simulink library "halout"  (R2021b)
settings: Solver=VariableStepAuto  StartTime=0.0  StopTime=10.0  RelTol=1e-3
undefined symbols (not defined in the file): C_TASK_5MS_S, FALSE, KHAL_CAN1FD1APS3E2E_flg, KHAL_CAN1FD1APS3TxReq_flg, KHAL_CAN1FD1VCU2E2E_flg, KHAL_CAN1FD1VCU2TxReq_flg, KHAL_CAN1FD1VCU3E2E_flg, KHAL_CAN1FD1VCU3TxReq_flg, KHAL_CAN1TxReq_flg, KHAL_CAN1VMCFCM1E2E_flg, KHAL_CAN1VMCFCM1TxReq_flg, KHAL_CAN2TxReq_flg, KHAL_CAN3FD3VCU1toNIDECTxReq_flg, KHAL_CAN3FD3VCU1TxReq_flg, KHAL_CAN3FD3VCU2E2E_flg, KHAL_CAN3FD3VCU2toNIDECE2E_flg, KHAL_CAN3FD3VCU2toNIDECTxReq_flg, KHAL_CAN3FD3VCU2TxReq_flg, KHAL_CAN3TxReq_flg, KHAL_CAN4FD4CE1000E2E_flg, KHAL_CAN4FD4CE1000TxReq_flg, KHAL_CAN4TxReq_flg, KHAL_CAN5TxReq_flg, KHAL_CAN6FD6APS3E2E_flg, KHAL_CAN6FD6APS3TxReq_flg, KHAL_CAN6FD6VCU2E2E_flg, KHAL_CAN6FD6VCU2TxReq_flg, KHAL_CAN6TxReq_flg, ONE_INT, TRUE, ZERO_INT
libraries: FVT_lib x500, simulink x235
(part 12 of 25)

== system halout/HAL_OUT/CAN4/FD4_CE200_0_0x217 ==
  BSCP_outputs : Inport  OutDataTypeStr=Bus: BSCP_outputs
  BOUTP_outputs : Inport  Port=2  OutDataTypeStr=Bus: BOUTP_outputs
  AmbLightBreath1 : Subsystem
  AmbLightBreath2 : Subsystem
  AmbLightBreath3 : Subsystem
  AmbLightBreath4 : Subsystem
  AmbLightBreath5 : Subsystem
  AmbLightBreath6 : Subsystem
  AmbLightBrightness1 : Subsystem
  AmbLightBrightness2 : Subsystem
  AmbLightBrightness3 : Subsystem
  AmbLightBrightness4 : Subsystem
  AmbLightBrightness5 : Subsystem
  AmbLightBrightness6 : Subsystem
  AmbLightColor1 : Subsystem
  AmbLightColor2 : Subsystem
  AmbLightColor3 : Subsystem
  AmbLightColor4 : Subsystem
  AmbLightColor5 : Subsystem
  AmbLightColor6 : Subsystem
  BCMBuzzerReq : Subsystem
  FDCBCMATCtrlCmd : Subsystem
  FDCBCMDimSw : Subsystem
  FDCBCMFWasSwSta : Subsystem
  FDCBCMFWipSwSta : Subsystem
  FDCBCMHazardINDCmd : Subsystem
  FDCBCMLockAlarmCmd : Subsystem
  FDCBCMPTGOpenHeightSta : Subsystem
  FDCBCMPassSWSta : Subsystem
  FDCBCMTurnSwSta : Subsystem
  FDCBCMTurnSwTSetStaSta : Subsystem
  FDCBCMUserHeightSetSta : Subsystem
  FDCBCMUserNowSta : Subsystem
  FDCDKCCommandToBCMCmd : Subsystem
  FDCDKCDKeyAreaPESta : Subsystem
  FDCDKCSPTGDetCmd : Subsystem
  FDCDKCSPTGOpenCmd : Subsystem
  FDCFGSAirIntCmd : Subsystem
  FDCFGSFGSChCmd : Subsystem
  FDCFGSFGSLearnCmd : Subsystem
  FDCFGSFuncStaCmd : Subsystem
  FDCFGSIONCmd : Subsystem
  FDCTHCMACTInitialCmd : Subsystem
  FDCTHCMAirIntZ3Sta : Subsystem
  FDHandleCmd : Subsystem
  FDLHandleLampCmd : Subsystem
  FDRHandleLampCmd : Subsystem
  Ground{,1..17} (18 alike) : Ground
  WelcomeLight : Subsystem
  bus_creator : BusCreator  Inputs=46  OutDataTypeStr=Bus: DT_CAN4_SG_FD4_CE200_0  NonVirtualBus=on
  bus_selector : BusSelector  OutputSignals=VOUTP_AmbLightBreath1_enum
  bus_selector1 : BusSelector  OutputSignals=VOUTP_AmbLightBreath2_enum
  bus_selector10 : BusSelector  OutputSignals=VOUTP_AmbLightBrightness5_enum
  bus_selector11 : BusSelector  OutputSignals=VOUTP_AmbLightBrightness6_enum
  bus_selector12 : BusSelector  OutputSignals=VOUTP_AmbLightColor1_enum
  bus_selector13 : BusSelector  OutputSignals=VOUTP_AmbLightColor2_enum
  bus_selector14 : BusSelector  OutputSignals=VOUTP_AmbLightColor3_enum
  bus_selector15 : BusSelector  OutputSignals=VOUTP_AmbLightColor4_enum
  bus_selector16 : BusSelector  OutputSignals=VOUTP_AmbLightColor5_enum
  bus_selector17 : BusSelector  OutputSignals=VOUTP_AmbLightColor6_enum
  bus_selector18 : BusSelector  OutputSignals=VOUTP_BCMBuzzerReq_flg
  bus_selector19 : BusSelector  OutputSignals=VOUTP_ATCtrl_enum
  bus_selector2 : BusSelector  OutputSignals=VOUTP_AmbLightBreath3_enum
  bus_selector20 : BusSelector  OutputSignals=VOUTP_DimSwSta_flg
  bus_selector21 : BusSelector  OutputSignals=VOUTP_FWasSwSta_enum
  bus_selector22 : BusSelector  OutputSignals=VOUTP_FWipSwSta_enum
  bus_selector23 : BusSelector  OutputSignals=VOUTP_HazardIND_flg
  bus_selector24 : BusSelector  OutputSignals=VOUTP_LockAlarm_enum
  bus_selector25 : BusSelector  OutputSignals=VOUTP_PassSWSta_flg
  bus_selector26 : BusSelector  OutputSignals=VOUTP_TurnSwSta_enum
  bus_selector27 : BusSelector  OutputSignals=VOUTP_UserNow_enum
  bus_selector3 : BusSelector  OutputSignals=VOUTP_AmbLightBreath4_enum
  bus_selector4 : BusSelector  OutputSignals=VOUTP_AmbLightBreath5_enum
  bus_selector5 : BusSelector  OutputSignals=VOUTP_AmbLightBreath6_enum
  bus_selector6 : BusSelector  OutputSignals=VOUTP_AmbLightBrightness1_enum
  bus_selector7 : BusSelector  OutputSignals=VOUTP_AmbLightBrightness2_enum
  bus_selector8 : BusSelector  OutputSignals=VOUTP_AmbLightBrightness3_enum
  bus_selector9 : BusSelector  OutputSignals=VOUTP_AmbLightBrightness4_enum
  FD4_CE200_0 : Outport
  wires:
  BSCP_outputs/1 -> [BSCP_outputs]
  BOUTP_outputs/1 -> [BOUTP_outputs]
  [CAN4_AmbLightBreath1] -> bus_creator/1  "CAN4_AmbLightBreath1"
  [CAN4_AmbLightBreath2] -> bus_creator/2  "CAN4_AmbLightBreath2"
  [CAN4_AmbLightBreath3] -> bus_creator/3  "CAN4_AmbLightBreath3"
  [CAN4_AmbLightBreath4] -> bus_creator/4  "CAN4_AmbLightBreath4"
  [CAN4_AmbLightBreath5] -> bus_creator/5  "CAN4_AmbLightBreath5"
  [CAN4_AmbLightBreath6] -> bus_creator/6  "CAN4_AmbLightBreath6"
  [CAN4_AmbLightBrightness1] -> bus_creator/7  "CAN4_AmbLightBrightness1"
  [CAN4_AmbLightBrightness2] -> bus_creator/8  "CAN4_AmbLightBrightness2"
  [CAN4_AmbLightBrightness3] -> bus_creator/9  "CAN4_AmbLightBrightness3"
  [CAN4_AmbLightBrightness4] -> bus_creator/10  "CAN4_AmbLightBrightness4"
  [CAN4_AmbLightBrightness5] -> bus_creator/11  "CAN4_AmbLightBrightness5"
  [CAN4_AmbLightBrightness6] -> bus_creator/12  "CAN4_AmbLightBrightness6"
  [CAN4_AmbLightColor1] -> bus_creator/13  "CAN4_AmbLightColor1"
  [CAN4_AmbLightColor2] -> bus_creator/14  "CAN4_AmbLightColor2"
  [CAN4_AmbLightColor3] -> bus_creator/15  "CAN4_AmbLightColor3"
  [CAN4_AmbLightColor4] -> bus_creator/16  "CAN4_AmbLightColor4"
  [CAN4_AmbLightColor5] -> bus_creator/17  "CAN4_AmbLightColor5"
  [CAN4_AmbLightColor6] -> bus_creator/18  "CAN4_AmbLightColor6"
  [CAN4_BCM_Buzzer_Req] -> bus_creator/19  "CAN4_BCM_Buzzer_Req"
  [CAN4_FDC_BCM_ATCtrl_Cmd] -> bus_creator/20  "CAN4_FDC_BCM_ATCtrl_Cmd"
  [CAN4_FDC_BCM_DimSw] -> bus_creator/21  "CAN4_FDC_BCM_DimSw"
  [CAN4_FDC_BCM_FWasSw_Sta] -> bus_creator/22  "CAN4_FDC_BCM_FWasSw_Sta"
  [CAN4_FDC_BCM_FWipSw_Sta] -> bus_creator/23  "CAN4_FDC_BCM_FWipSw_Sta"
  [CAN4_FDC_BCM_HazardIND_Cmd] -> bus_creator/24  "CAN4_FDC_BCM_HazardIND_Cmd"
  [CAN4_FDC_BCM_LockAlarm_Cmd] -> bus_creator/25  "CAN4_FDC_BCM_LockAlarm_Cmd"
  [CAN4_FDC_BCM_PTGOpenHeight_Sta] -> bus_creator/26  "CAN4_FDC_BCM_PTGOpenHeight_Sta"
  [CAN4_FDC_BCM_PassSW_Sta] -> bus_creator/27  "CAN4_FDC_BCM_PassSW_Sta"
  [CAN4_FDC_BCM_TurnSwTSetSta_Sta] -> bus_creator/28  "CAN4_FDC_BCM_TurnSwTSetSta_Sta"
  [CAN4_FDC_BCM_TurnSw_Sta] -> bus_creator/29  "CAN4_FDC_BCM_TurnSw_Sta"
  [CAN4_FDC_BCM_UserHeightSet_Sta] -> bus_creator/30  "CAN4_FDC_BCM_UserHeightSet_Sta"
  [CAN4_FDC_BCM_UserNow_Sta] -> bus_creator/31  "CAN4_FDC_BCM_UserNow_Sta"
  [CAN4_FDC_DKC_CommandToBCM_Cmd] -> bus_creator/32  "CAN4_FDC_DKC_CommandToBCM_Cmd"
  [CAN4_FDC_DKC_DKeyAreaPE_Sta] -> bus_creator/33  "CAN4_FDC_DKC_DKeyAreaPE_Sta"
  [CAN4_FDC_DKC_SPTGDet_Cmd] -> bus_creator/34  "CAN4_FDC_DKC_SPTGDet_Cmd"
  [CAN4_FDC_DKC_SPTGOpen_Cmd] -> bus_creator/35  "CAN4_FDC_DKC_SPTGOpen_Cmd"
  [CAN4_FDC_FGS_AirInt_Cmd] -> bus_creator/36  "CAN4_FDC_FGS_AirInt_Cmd"
  [CAN4_FDC_FGS_FGSCh_Cmd] -> bus_creator/37  "CAN4_FDC_FGS_FGSCh_Cmd"
  [CAN4_FDC_FGS_FGSLearn_Cmd] -> bus_creator/38  "CAN4_FDC_FGS_FGSLearn_Cmd"
  [CAN4_FDC_FGS_FuncSta_Cmd] -> bus_creator/39  "CAN4_FDC_FGS_FuncSta_Cmd"
  [CAN4_FDC_FGS_ION_Cmd] -> bus_creator/40  "CAN4_FDC_FGS_ION_Cmd"
  [CAN4_FDC_THCM_ACTInitial_Cmd] -> bus_creator/41  "CAN4_FDC_THCM_ACTInitial_Cmd"
  [CAN4_FDC_THCM_AirIntZ3_Sta] -> bus_creator/42  "CAN4_FDC_THCM_AirIntZ3_Sta"
  [CAN4_FDHandleCmd] -> bus_creator/43  "CAN4_FDHandleCmd"
  [CAN4_FDLHandleLampCmd] -> bus_creator/44  "CAN4_FDLHandleLampCmd"
  [CAN4_FDRHandleLampCmd] -> bus_creator/45  "CAN4_FDRHandleLampCmd"
  [CAN4_WelcomeLight] -> bus_creator/46  "CAN4_WelcomeLight"
  bus_creator/1 -> FD4_CE200_0/1
  AmbLightBreath1/1(CAN4_AmbLightBreath1) -> [CAN4_AmbLightBreath1]
  AmbLightBreath2/1(CAN4_AmbLightBreath2) -> [CAN4_AmbLightBreath2]
  AmbLightBreath3/1(CAN4_AmbLightBreath3) -> [CAN4_AmbLightBreath3]
  AmbLightBreath4/1(CAN4_AmbLightBreath4) -> [CAN4_AmbLightBreath4]
  AmbLightBreath5/1(CAN4_AmbLightBreath5) -> [CAN4_AmbLightBreath5]
  AmbLightBreath6/1(CAN4_AmbLightBreath6) -> [CAN4_AmbLightBreath6]
  AmbLightBrightness1/1(CAN4_AmbLightBrightness1) -> [CAN4_AmbLightBrightness1]
  AmbLightBrightness2/1(CAN4_AmbLightBrightness2) -> [CAN4_AmbLightBrightness2]
  AmbLightBrightness3/1(CAN4_AmbLightBrightness3) -> [CAN4_AmbLightBrightness3]
  AmbLightBrightness4/1(CAN4_AmbLightBrightness4) -> [CAN4_AmbLightBrightness4]
  AmbLightBrightness5/1(CAN4_AmbLightBrightness5) -> [CAN4_AmbLightBrightness5]
  AmbLightBrightness6/1(CAN4_AmbLightBrightness6) -> [CAN4_AmbLightBrightness6]
  AmbLightColor1/1(CAN4_AmbLightColor1) -> [CAN4_AmbLightColor1]
  AmbLightColor2/1(CAN4_AmbLightColor2) -> [CAN4_AmbLightColor2]
  AmbLightColor3/1(CAN4_AmbLightColor3) -> [CAN4_AmbLightColor3]
  AmbLightColor4/1(CAN4_AmbLightColor4) -> [CAN4_AmbLightColor4]
  AmbLightColor5/1(CAN4_AmbLightColor5) -> [CAN4_AmbLightColor5]
  AmbLightColor6/1(CAN4_AmbLightColor6) -> [CAN4_AmbLightColor6]
  BCMBuzzerReq/1(CAN4_BCM_Buzzer_Req) -> [CAN4_BCM_Buzzer_Req]
  FDCBCMATCtrlCmd/1(CAN4_FDC_BCM_ATCtrl_Cmd) -> [CAN4_FDC_BCM_ATCtrl_Cmd]
  FDCBCMDimSw/1(CAN4_FDC_BCM_DimSw) -> [CAN4_FDC_BCM_DimSw]
  FDCBCMFWasSwSta/1(CAN4_FDC_BCM_FWasSw_Sta) -> [CAN4_FDC_BCM_FWasSw_Sta]
  FDCBCMFWipSwSta/1(CAN4_FDC_BCM_FWipSw_Sta) -> [CAN4_FDC_BCM_FWipSw_Sta]
  FDCBCMHazardINDCmd/1(CAN4_FDC_BCM_HazardIND_Cmd) -> [CAN4_FDC_BCM_HazardIND_Cmd]
  FDCBCMLockAlarmCmd/1(CAN4_FDC_BCM_LockAlarm_Cmd) -> [CAN4_FDC_BCM_LockAlarm_Cmd]
  FDCBCMPTGOpenHeightSta/1(CAN4_FDC_BCM_PTGOpenHeight_Sta) -> [CAN4_FDC_BCM_PTGOpenHeight_Sta]
  FDCBCMPassSWSta/1(CAN4_FDC_BCM_PassSW_Sta) -> [CAN4_FDC_BCM_PassSW_Sta]
  FDCBCMTurnSwTSetStaSta/1(CAN4_FDC_BCM_TurnSwTSetSta_Sta) -> [CAN4_FDC_BCM_TurnSwTSetSta_Sta]
  FDCBCMTurnSwSta/1(CAN4_FDC_BCM_TurnSw_Sta) -> [CAN4_FDC_BCM_TurnSw_Sta]
  FDCBCMUserHeightSetSta/1(CAN4_FDC_BCM_UserHeightSet_Sta) -> [CAN4_FDC_BCM_UserHeightSet_Sta]
  FDCBCMUserNowSta/1(CAN4_FDC_BCM_UserNow_Sta) -> [CAN4_FDC_BCM_UserNow_Sta]
  FDCDKCCommandToBCMCmd/1(CAN4_FDC_DKC_CommandToBCM_Cmd) -> [CAN4_FDC_DKC_CommandToBCM_Cmd]
  FDCDKCDKeyAreaPESta/1(CAN4_FDC_DKC_DKeyAreaPE_Sta) -> [CAN4_FDC_DKC_DKeyAreaPE_Sta]
  FDCDKCSPTGDetCmd/1(CAN4_FDC_DKC_SPTGDet_Cmd) -> [CAN4_FDC_DKC_SPTGDet_Cmd]
  FDCDKCSPTGOpenCmd/1(CAN4_FDC_DKC_SPTGOpen_Cmd) -> [CAN4_FDC_DKC_SPTGOpen_Cmd]
  FDCFGSAirIntCmd/1(CAN4_FDC_FGS_AirInt_Cmd) -> [CAN4_FDC_FGS_AirInt_Cmd]
  FDCFGSFGSChCmd/1(CAN4_FDC_FGS_FGSCh_Cmd) -> [CAN4_FDC_FGS_FGSCh_Cmd]
  FDCFGSFGSLearnCmd/1(CAN4_FDC_FGS_FGSLearn_Cmd) -> [CAN4_FDC_FGS_FGSLearn_Cmd]
  FDCFGSFuncStaCmd/1(CAN4_FDC_FGS_FuncSta_Cmd) -> [CAN4_FDC_FGS_FuncSta_Cmd]
  FDCFGSIONCmd/1(CAN4_FDC_FGS_ION_Cmd) -> [CAN4_FDC_FGS_ION_Cmd]
  FDCTHCMACTInitialCmd/1(CAN4_FDC_THCM_ACTInitial_Cmd) -> [CAN4_FDC_THCM_ACTInitial_Cmd]
  FDCTHCMAirIntZ3Sta/1(CAN4_FDC_THCM_AirIntZ3_Sta) -> [CAN4_FDC_THCM_AirIntZ3_Sta]
  FDHandleCmd/1(CAN4_FDHandleCmd) -> [CAN4_FDHandleCmd]
  FDLHandleLampCmd/1(CAN4_FDLHandleLampCmd) -> [CAN4_FDLHandleLampCmd]
  FDRHandleLampCmd/1(CAN4_FDRHandleLampCmd) -> [CAN4_FDRHandleLampCmd]
  WelcomeLight/1(CAN4_WelcomeLight) -> [CAN4_WelcomeLight]
  bus_selector/1 -> AmbLightBreath1/1(AmbLightBreath1)  "<VOUTP_AmbLightBreath1_enum>"
  [BOUTP_outputs] -> bus_selector/1
  bus_selector1/1 -> AmbLightBreath2/1(AmbLightBreath2)  "<VOUTP_AmbLightBreath2_enum>"
  [BOUTP_outputs] -> bus_selector1/1
  bus_selector2/1 -> AmbLightBreath3/1(AmbLightBreath3)  "<VOUTP_AmbLightBreath3_enum>"
  [BOUTP_outputs] -> bus_selector2/1
  bus_selector3/1 -> AmbLightBreath4/1(AmbLightBreath4)  "<VOUTP_AmbLightBreath4_enum>"
  [BOUTP_outputs] -> bus_selector3/1
  bus_selector4/1 -> AmbLightBreath5/1(AmbLightBreath5)  "<VOUTP_AmbLightBreath5_enum>"
  [BOUTP_outputs] -> bus_selector4/1
  bus_selector5/1 -> AmbLightBreath6/1(AmbLightBreath6)  "<VOUTP_AmbLightBreath6_enum>"
  [BOUTP_outputs] -> bus_selector5/1
  bus_selector6/1 -> AmbLightBrightness1/1(AmbLightBrightness1)  "<VOUTP_AmbLightBrightness1_enum>"
  [BOUTP_outputs] -> bus_selector6/1
  bus_selector7/1 -> AmbLightBrightness2/1(AmbLightBrightness2)  "<VOUTP_AmbLightBrightness2_enum>"
  [BOUTP_outputs] -> bus_selector7/1
  bus_selector8/1 -> AmbLightBrightness3/1(AmbLightBrightness3)  "<VOUTP_AmbLightBrightness3_enum>"
  [BOUTP_outputs] -> bus_selector8/1
  bus_selector9/1 -> AmbLightBrightness4/1(AmbLightBrightness4)  "<VOUTP_AmbLightBrightness4_enum>"
  [BOUTP_outputs] -> bus_selector9/1
  bus_selector10/1 -> AmbLightBrightness5/1(AmbLightBrightness5)  "<VOUTP_AmbLightBrightness5_enum>"
  [BOUTP_outputs] -> bus_selector10/1
  bus_selector11/1 -> AmbLightBrightness6/1(AmbLightBrightness6)  "<VOUTP_AmbLightBrightness6_enum>"
  [BOUTP_outputs] -> bus_selector11/1
  bus_selector12/1 -> AmbLightColor1/1(AmbLightColor1)  "<VOUTP_AmbLightColor1_enum>"
  [BOUTP_outputs] -> bus_selector12/1
  bus_selector13/1 -> AmbLightColor2/1(AmbLightColor2)  "<VOUTP_AmbLightColor2_enum>"
  [BOUTP_outputs] -> bus_selector13/1
  bus_selector14/1 -> AmbLightColor3/1(AmbLightColor3)  "<VOUTP_AmbLightColor3_enum>"
  [BOUTP_outputs] -> bus_selector14/1
  bus_selector15/1 -> AmbLightColor4/1(AmbLightColor4)  "<VOUTP_AmbLightColor4_enum>"
  [BOUTP_outputs] -> bus_selector15/1
  bus_selector16/1 -> AmbLightColor5/1(AmbLightColor5)  "<VOUTP_AmbLightColor5_enum>"
  [BOUTP_outputs] -> bus_selector16/1
  bus_selector17/1 -> AmbLightColor6/1(AmbLightColor6)  "<VOUTP_AmbLightColor6_enum>"
  [BOUTP_outputs] -> bus_selector17/1
  bus_selector18/1 -> BCMBuzzerReq/1(BCMBuzzerReq)  "<VOUTP_BCMBuzzerReq_flg>"
  [BOUTP_outputs] -> bus_selector18/1
  bus_selector19/1 -> FDCBCMATCtrlCmd/1(FDCBCMATCtrlCmd)  "<VOUTP_ATCtrl_enum>"
  [BOUTP_outputs] -> bus_selector19/1
  bus_selector20/1 -> FDCBCMDimSw/1(FDCBCMDimSw)  "<VOUTP_DimSwSta_flg>"
  [BOUTP_outputs] -> bus_selector20/1
  bus_selector21/1 -> FDCBCMFWasSwSta/1(FDCBCMFWasSwSta)  "<VOUTP_FWasSwSta_enum>"
  [BOUTP_outputs] -> bus_selector21/1
  bus_selector22/1 -> FDCBCMFWipSwSta/1(FDCBCMFWipSwSta)  "<VOUTP_FWipSwSta_enum>"
  [BOUTP_outputs] -> bus_selector22/1
  bus_selector23/1 -> FDCBCMHazardINDCmd/1(FDCBCMHazardINDCmd)  "<VOUTP_HazardIND_flg>"
  [BOUTP_outputs] -> bus_selector23/1
  bus_selector24/1 -> FDCBCMLockAlarmCmd/1(FDCBCMLockAlarmCmd)  "<VOUTP_LockAlarm_enum>"
  [BOUTP_outputs] -> bus_selector24/1
  Ground/1 -> FDCBCMPTGOpenHeightSta/1(FDCBCMPTGOpenHeightSta)
  bus_selector25/1 -> FDCBCMPassSWSta/1(FDCBCMPassSWSta)  "<VOUTP_PassSWSta_flg>"
  [BOUTP_outputs] -> bus_selector25/1
  Ground1/1 -> FDCBCMTurnSwTSetStaSta/1(FDCBCMTurnSwTSetStaSta)
  bus_selector26/1 -> FDCBCMTurnSwSta/1(FDCBCMTurnSwSta)  "<VOUTP_TurnSwSta_enum>"
  [BOUTP_outputs] -> bus_selector26/1
  Ground2/1 -> FDCBCMUserHeightSetSta/1(FDCBCMUserHeightSetSta)
  bus_selector27/1 -> FDCBCMUserNowSta/1(FDCBCMUserNowSta)  "<VOUTP_UserNow_enum>"
  [BOUTP_outputs] -> bus_selector27/1
  Ground3/1 -> FDCDKCCommandToBCMCmd/1(FDCDKCCommandToBCMCmd)
  Ground4/1 -> FDCDKCDKeyAreaPESta/1(FDCDKCDKeyAreaPESta)
  Ground5/1 -> FDCDKCSPTGDetCmd/1(FDCDKCSPTGDetCmd)
  Ground6/1 -> FDCDKCSPTGOpenCmd/1(FDCDKCSPTGOpenCmd)
  Ground7/1 -> FDCFGSAirIntCmd/1(FDCFGSAirIntCmd)
  Ground8/1 -> FDCFGSFGSChCmd/1(FDCFGSFGSChCmd)
  Ground9/1 -> FDCFGSFGSLearnCmd/1(FDCFGSFGSLearnCmd)
  Ground10/1 -> FDCFGSFuncStaCmd/1(FDCFGSFuncStaCmd)
  Ground11/1 -> FDCFGSIONCmd/1(FDCFGSIONCmd)
  Ground12/1 -> FDCTHCMACTInitialCmd/1(FDCTHCMACTInitialCmd)
  Ground13/1 -> FDCTHCMAirIntZ3Sta/1(FDCTHCMAirIntZ3Sta)
  Ground14/1 -> FDHandleCmd/1(FDHandleCmd)
  Ground15/1 -> FDLHandleLampCmd/1(FDLHandleLampCmd)
  Ground16/1 -> FDRHandleLampCmd/1(FDRHandleLampCmd)
  Ground17/1 -> WelcomeLight/1(WelcomeLight)

== system halout/HAL_OUT/CAN4/Function-Call Subsystem ==
  function : TriggerPort  TriggerType=function-call  VariantControl=(inherit)
  Add : Sum
  Constant : Constant  Value=ONE_INT
  Constant1 : Constant  Value=ZERO_INT
  Constant2 : Constant  Value=uint8(10)
  GreaterThan : RelationalOperator  Operator=>  OutDataTypeStr=boolean  RndMeth=Simplest
  Switch : Switch  Criteria=u2 ~= 0
  Unit Delay : UnitDelay  SampleTime=-1  HasFrameUpgradeWarning=on
  TriggerCAN4VCU1_CNT : Outport
  wires:
  Add/1 -> Switch/3, GreaterThan/1
  Unit Delay/1 -> Add/1
  Constant/1 -> Add/2
  Switch/1 -> TriggerCAN4VCU1_CNT/1, Unit Delay/1
  Constant2/1 -> GreaterThan/2
  GreaterThan/1 -> Switch/2
  Constant1/1 -> Switch/1

== system halout/HAL_OUT/CAN4/GW4_CE100_0_0x253 ==
  BSCP_outputs : Inport  OutDataTypeStr=Bus: BSCP_outputs
  BOUTP_outputs : Inport  Port=2  OutDataTypeStr=Bus: BOUTP_outputs
  FDCPTGinnerSW2 : Subsystem
  LDrvCtrlCmd : Subsystem
  LPasCtrlCmd : Subsystem
  LRLDCtrlCmd : Subsystem
  LRRDCtrlCmd : Subsystem
  bus_creator : BusCreator  Inputs=5  OutDataTypeStr=Bus: DT_CAN4_SG_GW4_CE100_0  NonVirtualBus=on
  bus_selector : BusSelector  OutputSignals=VOUTP_PTGInnerSW2_enum
  bus_selector1 : BusSelector  OutputSignals=VOUTP_LDrvCtrlCmd_pct
  bus_selector2 : BusSelector  OutputSignals=VOUTP_LPasCtrlCmd_pct
  bus_selector3 : BusSelector  OutputSignals=VOUTP_LRLDCtrlCmd_pct
  bus_selector4 : BusSelector  OutputSignals=VOUTP_LRRDCtrlCmd_pct
  GW4_CE100_0 : Outport
  wires:
  BSCP_outputs/1 -> [BSCP_outputs]
  BOUTP_outputs/1 -> [BOUTP_outputs]
  [CAN4_FDC_PTG_inner_SW_2] -> bus_creator/1  "CAN4_FDC_PTG_inner_SW_2"
  [CAN4_L_Drv_CtrlCmd] -> bus_creator/2  "CAN4_L_Drv_CtrlCmd"
  [CAN4_L_Pas_CtrlCmd] -> bus_creator/3  "CAN4_L_Pas_CtrlCmd"
  [CAN4_L_RLD_CtrlCmd] -> bus_creator/4  "CAN4_L_RLD_CtrlCmd"
  [CAN4_L_RRD_CtrlCmd] -> bus_creator/5  "CAN4_L_RRD_CtrlCmd"
  bus_creator/1 -> GW4_CE100_0/1
  FDCPTGinnerSW2/1(CAN4_FDC_PTG_inner_SW_2) -> [CAN4_FDC_PTG_inner_SW_2]
  LDrvCtrlCmd/1(CAN4_L_Drv_CtrlCmd) -> [CAN4_L_Drv_CtrlCmd]
  LPasCtrlCmd/1(CAN4_L_Pas_CtrlCmd) -> [CAN4_L_Pas_CtrlCmd]
  LRLDCtrlCmd/1(CAN4_L_RLD_CtrlCmd) -> [CAN4_L_RLD_CtrlCmd]
  LRRDCtrlCmd/1(CAN4_L_RRD_CtrlCmd) -> [CAN4_L_RRD_CtrlCmd]
  bus_selector/1 -> FDCPTGinnerSW2/1(FDCPTGinnerSW2)  "<VOUTP_PTGInnerSW2_enum>"
  [BOUTP_outputs] -> bus_selector/1
  bus_selector1/1 -> LDrvCtrlCmd/1(LDrvCtrlCmd)  "<VOUTP_LDrvCtrlCmd_pct>"
  [BOUTP_outputs] -> bus_selector1/1
  bus_selector2/1 -> LPasCtrlCmd/1(LPasCtrlCmd)  "<VOUTP_LPasCtrlCmd_pct>"
  [BOUTP_outputs] -> bus_selector2/1
  bus_selector3/1 -> LRLDCtrlCmd/1(LRLDCtrlCmd)  "<VOUTP_LRLDCtrlCmd_pct>"
  [BOUTP_outputs] -> bus_selector3/1
  bus_selector4/1 -> LRRDCtrlCmd/1(LRRDCtrlCmd)  "<VOUTP_LRRDCtrlCmd_pct>"
  [BOUTP_outputs] -> bus_selector4/1

== system halout/HAL_OUT/CAN5/FD5_CE100_0_0x118 ==
  BSCP_outputs : Inport  OutDataTypeStr=Bus: BSCP_outputs
  BOUTP_outputs : Inport  Port=2  OutDataTypeStr=Bus: BOUTP_outputs
  AllDoorSW : Subsystem
  AntitheftSta : Subsystem
  BCMDoorLockSta : Subsystem
  CCUACLampSts : Subsystem
  CCUCbnPreACWkSts : Subsystem
  CCUCbnPreEstimdTi : Subsystem
  CCUCbnPreSts : Subsystem
  FDTBOXDTCDataErr : Subsystem
  FDTBOXDTCDataSta : Subsystem
  FDTBOXVehDataErr : Subsystem
  FDTBOXVehDataSta : Subsystem
  Ground{,1..7} (8 alike) : Ground
  HoodSW : Subsystem
  LowSOCWarn : Subsystem
  PwrSta : Subsystem
  ReVehThdChkSta : Subsystem
  ShiftGearPosn : Subsystem
  TCountSta : Subsystem
  TailgateRemote : Subsystem
  TailgateSW : Subsystem
  VehMalfunLevel : Subsystem
  bus_creator : BusCreator  Inputs=20  OutDataTypeStr=Bus: DT_CAN5_SG_FD5_CE100_0  NonVirtualBus=on
  bus_selector : BusSelector  OutputSignals=VOUTP_AllDoorSW_flg
  bus_selector1 : BusSelector  OutputSignals=VOUTP_AntitheftSta_enum
  bus_selector10 : BusSelector  OutputSignals=VOUTP_TailgateRemote_enum
  bus_selector11 : BusSelector  OutputSignals=VOUTP_TailgateSW_flg
  bus_selector2 : BusSelector  OutputSignals=VOUTP_BCMDoorLockSta_flg
  bus_selector3 : BusSelector  OutputSignals=VOUTP_CCUACLampSts_flg
  bus_selector4 : BusSelector  OutputSignals=VOUTP_HoodSW_flg
  bus_selector5 : BusSelector  OutputSignals=VOUTP_LowSOCWarn_enum
  bus_selector6 : BusSelector  OutputSignals=VOUTP_PowerSta_enum
  bus_selector7 : BusSelector  OutputSignals=VOUTP_ReVehThdChkSta_enum
  bus_selector8 : BusSelector  OutputSignals=VOUTP_ShiftGearPosn_enum
  bus_selector9 : BusSelector  OutputSignals=VOUTP_TCountSta_enum
  FD5_CE100_0 : Outport
  wires:
  BSCP_outputs/1 -> [BSCP_outputs]
  BOUTP_outputs/1 -> [BOUTP_outputs]
  [CAN5_AllDoorSW] -> bus_creator/1  "CAN5_AllDoorSW"
  [CAN5_AntitheftSta] -> bus_creator/2  "CAN5_AntitheftSta"
  [CAN5_BCM_DoorLock_Sta] -> bus_creator/3  "CAN5_BCM_DoorLock_Sta"
  [CAN5_CCU_ACLampSts] -> bus_creator/4  "CAN5_CCU_ACLampSts"
  [CAN5_CCU_CbnPreACWkSts] -> bus_creator/5  "CAN5_CCU_CbnPreACWkSts"
  [CAN5_CCU_CbnPreEstimdTi] -> bus_creator/6  "CAN5_CCU_CbnPreEstimdTi"
  [CAN5_CCU_CbnPreSts] -> bus_creator/7  "CAN5_CCU_CbnPreSts"
  [CAN5_FD_TBOX_DTCData_Err] -> bus_creator/8  "CAN5_FD_TBOX_DTCData_Err"
  [CAN5_FD_TBOX_DTCData_Sta] -> bus_creator/9  "CAN5_FD_TBOX_DTCData_Sta"
  [CAN5_FD_TBOX_VehData_Err] -> bus_creator/10  "CAN5_FD_TBOX_VehData_Err"
  [CAN5_FD_TBOX_VehData_Sta] -> bus_creator/11  "CAN5_FD_TBOX_VehData_Sta"
  [CAN5_HoodSW] -> bus_creator/12  "CAN5_HoodSW"
  [CAN5_LowSOCWarn] -> bus_creator/13  "CAN5_LowSOCWarn"
  [CAN5_PwrSta] -> bus_creator/14  "CAN5_PwrSta"
  [CAN5_Re_VehThdChkSta] -> bus_creator/15  "CAN5_Re_VehThdChkSta"
  [CAN5_ShiftGearPosn] -> bus_creator/16  "CAN5_ShiftGearPosn"
  [CAN5_TCountSta] -> bus_creator/17  "CAN5_TCountSta"
  [CAN5_TailgateRemote] -> bus_creator/18  "CAN5_TailgateRemote"
  [CAN5_Tailgate_SW] -> bus_creator/19  "CAN5_Tailgate_SW"
  [CAN5_VehMalfunLevel] -> bus_creator/20  "CAN5_VehMalfunLevel"
  bus_creator/1 -> FD5_CE100_0/1
  AllDoorSW/1(CAN5_AllDoorSW) -> [CAN5_AllDoorSW]
  AntitheftSta/1(CAN5_AntitheftSta) -> [CAN5_AntitheftSta]
  BCMDoorLockSta/1(CAN5_BCM_DoorLock_Sta) -> [CAN5_BCM_DoorLock_Sta]
  CCUACLampSts/1(CAN5_CCU_ACLampSts) -> [CAN5_CCU_ACLampSts]
  CCUCbnPreACWkSts/1(CAN5_CCU_CbnPreACWkSts) -> [CAN5_CCU_CbnPreACWkSts]
  CCUCbnPreEstimdTi/1(CAN5_CCU_CbnPreEstimdTi) -> [CAN5_CCU_CbnPreEstimdTi]
  CCUCbnPreSts/1(CAN5_CCU_CbnPreSts) -> [CAN5_CCU_CbnPreSts]
  FDTBOXDTCDataErr/1(CAN5_FD_TBOX_DTCData_Err) -> [CAN5_FD_TBOX_DTCData_Err]
  FDTBOXDTCDataSta/1(CAN5_FD_TBOX_DTCData_Sta) -> [CAN5_FD_TBOX_DTCData_Sta]
  FDTBOXVehDataErr/1(CAN5_FD_TBOX_VehData_Err) -> [CAN5_FD_TBOX_VehData_Err]
  FDTBOXVehDataSta/1(CAN5_FD_TBOX_VehData_Sta) -> [CAN5_FD_TBOX_VehData_Sta]
  HoodSW/1(CAN5_HoodSW) -> [CAN5_HoodSW]
  LowSOCWarn/1(CAN5_LowSOCWarn) -> [CAN5_LowSOCWarn]
  PwrSta/1(CAN5_PwrSta) -> [CAN5_PwrSta]
  ReVehThdChkSta/1(CAN5_Re_VehThdChkSta) -> [CAN5_Re_VehThdChkSta]
  ShiftGearPosn/1(CAN5_ShiftGearPosn) -> [CAN5_ShiftGearPosn]
  TCountSta/1(CAN5_TCountSta) -> [CAN5_TCountSta]
  TailgateRemote/1(CAN5_TailgateRemote) -> [CAN5_TailgateRemote]
  TailgateSW/1(CAN5_Tailgate_SW) -> [CAN5_Tailgate_SW]
  VehMalfunLevel/1(CAN5_VehMalfunLevel) -> [CAN5_VehMalfunLevel]
  bus_selector/1 -> AllDoorSW/1(AllDoorSW)  "<VOUTP_AllDoorSW_flg>"
  [BOUTP_outputs] -> bus_selector/1
  bus_selector1/1 -> AntitheftSta/1(AntitheftSta)  "<VOUTP_AntitheftSta_enum>"
  [BOUTP_outputs] -> bus_selector1/1
  bus_selector2/1 -> BCMDoorLockSta/1(BCMDoorLockSta)  "<VOUTP_BCMDoorLockSta_flg>"
  [BOUTP_outputs] -> bus_selector2/1
  bus_selector3/1 -> CCUACLampSts/1(CCUACLampSts)  "<VOUTP_CCUACLampSts_flg>"
  [BOUTP_outputs] -> bus_selector3/1
  Ground/1 -> CCUCbnPreACWkSts/1(CCUCbnPreACWkSts)
  Ground1/1 -> CCUCbnPreEstimdTi/1(CCUCbnPreEstimdTi)
  Ground2/1 -> CCUCbnPreSts/1(CCUCbnPreSts)
  Ground3/1 -> FDTBOXDTCDataErr/1(FDTBOXDTCDataErr)
  Ground4/1 -> FDTBOXDTCDataSta/1(FDTBOXDTCDataSta)
  Ground5/1 -> FDTBOXVehDataErr/1(FDTBOXVehDataErr)
  Ground6/1 -> FDTBOXVehDataSta/1(FDTBOXVehDataSta)
  bus_selector4/1 -> HoodSW/1(HoodSW)  "<VOUTP_HoodSW_flg>"
  [BOUTP_outputs] -> bus_selector4/1
  bus_selector5/1 -> LowSOCWarn/1(LowSOCWarn)  "<VOUTP_LowSOCWarn_enum>"
  [BOUTP_outputs] -> bus_selector5/1
  bus_selector6/1 -> PwrSta/1(PwrSta)  "<VOUTP_PowerSta_enum>"
  [BOUTP_outputs] -> bus_selector6/1
  bus_selector7/1 -> ReVehThdChkSta/1(ReVehThdChkSta)  "<VOUTP_ReVehThdChkSta_enum>"
  [BOUTP_outputs] -> bus_selector7/1
  bus_selector8/1 -> ShiftGearPosn/1(ShiftGearPosn)  "<VOUTP_ShiftGearPosn_enum>"
  [BOUTP_outputs] -> bus_selector8/1
  bus_selector9/1 -> TCountSta/1(TCountSta)  "<VOUTP_TCountSta_enum>"
  [BOUTP_outputs] -> bus_selector9/1
  bus_selector10/1 -> TailgateRemote/1(TailgateRemote)  "<VOUTP_TailgateRemote_enum>"
  [BOUTP_outputs] -> bus_selector10/1
  bus_selector11/1 -> TailgateSW/1(TailgateSW)  "<VOUTP_TailgateSW_flg>"
  [BOUTP_outputs] -> bus_selector11/1
  Ground7/1 -> VehMalfunLevel/1(VehMalfunLevel)

== system halout/HAL_OUT/CAN5/FD5_Debug1_0x4D0 ==
  BSCP_outputs : Inport  OutDataTypeStr=Bus: BSCP_outputs
  BOUTP_outputs : Inport  Port=2  OutDataTypeStr=Bus: BOUTP_outputs
  ID1ALTU : Subsystem
  ID1LocALTU : Subsystem
  ID1messageALTU : Subsystem
  ID2ALTU : Subsystem
  ID2LocALTU : Subsystem
  ID2messageALTU : Subsystem
  ID3ALTU : Subsystem
  ID3LocALTU : Subsystem
  ID3messageALTU : Subsystem
  ID4ALTU : Subsystem
  ID4LocALTU : Subsystem
  ID4messageALTU : Subsystem
  IDinALTU : Subsystem
  LFSensorMode : Subsystem
  LRSensorMode : Subsystem
  RFFATALTU : Subsystem
  RFSensorMode : Subsystem
  RRSensorMode : Subsystem
  S1WheelDebugALTU : Subsystem
  S2WheelDebugALTU : Subsystem
  S3WheelDebugALTU : Subsystem
  S4WheelDebugALTU : Subsystem
  bus_creator : BusCreator  Inputs=22  OutDataTypeStr=Bus: DT_CAN5_SG_FD5_Debug1  NonVirtualBus=on
  bus_selector : BusSelector  OutputSignals=VOUTP_S1ID_raw32
  bus_selector1 : BusSelector  OutputSignals=VOUTP_S1L_enum
  bus_selector10 : BusSelector  OutputSignals=VOUTP_S4L_enum
  bus_selector11 : BusSelector  OutputSignals=VOUTP_ID4messageALTU_raw8
  bus_selector12 : BusSelector  OutputSignals=VOUTP_IDin_raw32
  bus_selector13 : BusSelector  OutputSignals=VOUTP_LFSensorMode_flg
  bus_selector14 : BusSelector  OutputSignals=VOUTP_LRSensorMode_flg
  bus_selector15 : BusSelector  OutputSignals=VOUTP_RFSensorMode_flg
  bus_selector16 : BusSelector  OutputSignals=VOUTP_FAT_flg
  bus_selector17 : BusSelector  OutputSignals=VOUTP_RRSensorMode_flg
  bus_selector18 : BusSelector  OutputSignals=VOUTP_S1WheelDebugALTU_pct
  bus_selector19 : BusSelector  OutputSignals=VOUTP_S2WheelDebugALTU_pct
  bus_selector2 : BusSelector  OutputSignals=VOUTP_ID1messageALTU_raw8
  bus_selector20 : BusSelector  OutputSignals=VOUTP_S3WheelDebugALTU_pct
  bus_selector21 : BusSelector  OutputSignals=VOUTP_S4WheelDebugALTU_pct
  bus_selector3 : BusSelector  OutputSignals=VOUTP_S2ID_raw32
  bus_selector4 : BusSelector  OutputSignals=VOUTP_S2L_enum
  bus_selector5 : BusSelector  OutputSignals=VOUTP_ID2messageALTU_raw8
  bus_selector6 : BusSelector  OutputSignals=VOUTP_S3ID_raw32
  bus_selector7 : BusSelector  OutputSignals=VOUTP_S3L_enum
  bus_selector8 : BusSelector  OutputSignals=VOUTP_ID3messageALTU_raw8
  bus_selector9 : BusSelector  OutputSignals=VOUTP_S4ID_raw32
  FD5_Debug1 : Outport
  wires:
  BSCP_outputs/1 -> [BSCP_outputs]
  BOUTP_outputs/1 -> [BOUTP_outputs]
  [CAN5_ID1_ALTU] -> bus_creator/1  "CAN5_ID1_ALTU"
  [CAN5_ID1_Loc_ALTU] -> bus_creator/2  "CAN5_ID1_Loc_ALTU"
  [CAN5_ID1_message_ALTU] -> bus_creator/3  "CAN5_ID1_message_ALTU"
  [CAN5_ID2_ALTU] -> bus_creator/4  "CAN5_ID2_ALTU"
  [CAN5_ID2_Loc_ALTU] -> bus_creator/5  "CAN5_ID2_Loc_ALTU"
  [CAN5_ID2_message_ALTU] -> bus_creator/6  "CAN5_ID2_message_ALTU"
  [CAN5_ID3_ALTU] -> bus_creator/7  "CAN5_ID3_ALTU"
  [CAN5_ID3_Loc_ALTU] -> bus_creator/8  "CAN5_ID3_Loc_ALTU"
  [CAN5_ID3_message_ALTU] -> bus_creator/9  "CAN5_ID3_message_ALTU"
  [CAN5_ID4_ALTU] -> bus_creator/10  "CAN5_ID4_ALTU"
  [CAN5_ID4_Loc_ALTU] -> bus_creator/11  "CAN5_ID4_Loc_ALTU"
  [CAN5_ID4_message_ALTU] -> bus_creator/12  "CAN5_ID4_message_ALTU"
  [CAN5_IDin_ALTU] -> bus_creator/13  "CAN5_IDin_ALTU"
  [CAN5_LFSensorMode] -> bus_creator/14  "CAN5_LFSensorMode"
  [CAN5_LRSensorMode] -> bus_creator/15  "CAN5_LRSensorMode"
  [CAN5_RFSensorMode] -> bus_creator/16  "CAN5_RFSensorMode"
  [CAN5_RF_FAT_ALTU] -> bus_creator/17  "CAN5_RF_FAT_ALTU"
  [CAN5_RRSensorMode] -> bus_creator/18  "CAN5_RRSensorMode"
  [CAN5_S1WheelDebug_ALTU] -> bus_creator/19  "CAN5_S1WheelDebug_ALTU"
  [CAN5_S2WheelDebug_ALTU] -> bus_creator/20  "CAN5_S2WheelDebug_ALTU"
  [CAN5_S3WheelDebug_ALTU] -> bus_creator/21  "CAN5_S3WheelDebug_ALTU"
  [CAN5_S4WheelDebug_ALTU] -> bus_creator/22  "CAN5_S4WheelDebug_ALTU"
  bus_creator/1 -> FD5_Debug1/1
  ID1ALTU/1(CAN5_ID1_ALTU) -> [CAN5_ID1_ALTU]
  ID1LocALTU/1(CAN5_ID1_Loc_ALTU) -> [CAN5_ID1_Loc_ALTU]
  ID1messageALTU/1(CAN5_ID1_message_ALTU) -> [CAN5_ID1_message_ALTU]
  ID2ALTU/1(CAN5_ID2_ALTU) -> [CAN5_ID2_ALTU]
  ID2LocALTU/1(CAN5_ID2_Loc_ALTU) -> [CAN5_ID2_Loc_ALTU]
  ID2messageALTU/1(CAN5_ID2_message_ALTU) -> [CAN5_ID2_message_ALTU]
  ID3ALTU/1(CAN5_ID3_ALTU) -> [CAN5_ID3_ALTU]
  ID3LocALTU/1(CAN5_ID3_Loc_ALTU) -> [CAN5_ID3_Loc_ALTU]
  ID3messageALTU/1(CAN5_ID3_message_ALTU) -> [CAN5_ID3_message_ALTU]
  ID4ALTU/1(CAN5_ID4_ALTU) -> [CAN5_ID4_ALTU]
  ID4LocALTU/1(CAN5_ID4_Loc_ALTU) -> [CAN5_ID4_Loc_ALTU]
  ID4messageALTU/1(CAN5_ID4_message_ALTU) -> [CAN5_ID4_message_ALTU]
  IDinALTU/1(CAN5_IDin_ALTU) -> [CAN5_IDin_ALTU]
  LFSensorMode/1(CAN5_LFSensorMode) -> [CAN5_LFSensorMode]
  LRSensorMode/1(CAN5_LRSensorMode) -> [CAN5_LRSensorMode]
  RFSensorMode/1(CAN5_RFSensorMode) -> [CAN5_RFSensorMode]
  RFFATALTU/1(CAN5_RF_FAT_ALTU) -> [CAN5_RF_FAT_ALTU]
  RRSensorMode/1(CAN5_RRSensorMode) -> [CAN5_RRSensorMode]
  S1WheelDebugALTU/1(CAN5_S1WheelDebug_ALTU) -> [CAN5_S1WheelDebug_ALTU]
  S2WheelDebugALTU/1(CAN5_S2WheelDebug_ALTU) -> [CAN5_S2WheelDebug_ALTU]
  S3WheelDebugALTU/1(CAN5_S3WheelDebug_ALTU) -> [CAN5_S3WheelDebug_ALTU]
  S4WheelDebugALTU/1(CAN5_S4WheelDebug_ALTU) -> [CAN5_S4WheelDebug_ALTU]
  bus_selector/1 -> ID1ALTU/1(ID1ALTU)  "<VOUTP_S1ID_raw32>"
  [BOUTP_outputs] -> bus_selector/1
  bus_selector1/1 -> ID1LocALTU/1(ID1LocALTU)  "<VOUTP_S1L_enum>"
  [BOUTP_outputs] -> bus_selector1/1
  bus_selector2/1 -> ID1messageALTU/1(ID1messageALTU)  "<VOUTP_ID1messageALTU_raw8>"
  [BOUTP_outputs] -> bus_selector2/1
  bus_selector3/1 -> ID2ALTU/1(ID2ALTU)  "<VOUTP_S2ID_raw32>"
  [BOUTP_outputs] -> bus_selector3/1
  bus_selector4/1 -> ID2LocALTU/1(ID2LocALTU)  "<VOUTP_S2L_enum>"
  [BOUTP_outputs] -> bus_selector4/1
  bus_selector5/1 -> ID2messageALTU/1(ID2messageALTU)  "<VOUTP_ID2messageALTU_raw8>"
  [BOUTP_outputs] -> bus_selector5/1
  bus_selector6/1 -> ID3ALTU/1(ID3ALTU)  "<VOUTP_S3ID_raw32>"
  [BOUTP_outputs] -> bus_selector6/1
  bus_selector7/1 -> ID3LocALTU/1(ID3LocALTU)  "<VOUTP_S3L_enum>"
  [BOUTP_outputs] -> bus_selector7/1
  bus_selector8/1 -> ID3messageALTU/1(ID3messageALTU)  "<VOUTP_ID3messageALTU_raw8>"
  [BOUTP_outputs] -> bus_selector8/1
  bus_selector9/1 -> ID4ALTU/1(ID4ALTU)  "<VOUTP_S4ID_raw32>"
  [BOUTP_outputs] -> bus_selector9/1
  bus_selector10/1 -> ID4LocALTU/1(ID4LocALTU)  "<VOUTP_S4L_enum>"
  [BOUTP_outputs] -> bus_selector10/1
  bus_selector11/1 -> ID4messageALTU/1(ID4messageALTU)  "<VOUTP_ID4messageALTU_raw8>"
  [BOUTP_outputs] -> bus_selector11/1
  bus_selector12/1 -> IDinALTU/1(IDinALTU)  "<VOUTP_IDin_raw32>"
  [BOUTP_outputs] -> bus_selector12/1
  bus_selector13/1 -> LFSensorMode/1(LFSensorMode)  "<VOUTP_LFSensorMode_flg>"
  [BOUTP_outputs] -> bus_selector13/1
  bus_selector14/1 -> LRSensorMode/1(LRSensorMode)  "<VOUTP_LRSensorMode_flg>"
  [BOUTP_outputs] -> bus_selector14/1
  bus_selector15/1 -> RFSensorMode/1(RFSensorMode)  "<VOUTP_RFSensorMode_flg>"
  [BOUTP_outputs] -> bus_selector15/1
  bus_selector16/1 -> RFFATALTU/1(RFFATALTU)  "<VOUTP_FAT_flg>"
  [BOUTP_outputs] -> bus_selector16/1
  bus_selector17/1 -> RRSensorMode/1(RRSensorMode)  "<VOUTP_RRSensorMode_flg>"
  [BOUTP_outputs] -> bus_selector17/1
  bus_selector18/1 -> S1WheelDebugALTU/1(S1WheelDebugALTU)  "<VOUTP_S1WheelDebugALTU_pct>"
  [BOUTP_outputs] -> bus_selector18/1
  bus_selector19/1 -> S2WheelDebugALTU/1(S2WheelDebugALTU)  "<VOUTP_S2WheelDebugALTU_pct>"
  [BOUTP_outputs] -> bus_selector19/1
  bus_selector20/1 -> S3WheelDebugALTU/1(S3WheelDebugALTU)  "<VOUTP_S3WheelDebugALTU_pct>"
  [BOUTP_outputs] -> bus_selector20/1
  bus_selector21/1 -> S4WheelDebugALTU/1(S4WheelDebugALTU)  "<VOUTP_S4WheelDebugALTU_pct>"
  [BOUTP_outputs] -> bus_selector21/1

== system halout/HAL_OUT/CAN6/FD6_APS3_0x238 ==
  BSCP_outputs : Inport  OutDataTypeStr=Bus: BSCP_outputs
  BOUTP_outputs : Inport  Port=2  OutDataTypeStr=Bus: BOUTP_outputs
  Trigger : TriggerPort  TriggerType=function-call  VariantControl=(inherit)
  APS3LifeCount : Subsystem
  APS3checksum : Subsystem
  APSAngleTarget : Subsystem
  APSDecReq : Subsystem
  APSDecReqA : Subsystem
  APSOpenPTG : Subsystem
  APSReq : Subsystem
  APSRqEPSCtrl : Subsystem
  APSStaSystem : Subsystem
  APSVRqEPSCtrl : Subsystem
  Byte_0 : Subsystem
  Byte_1 : Subsystem
  Byte_{8..15} (8 alike) : Constant  Value=ZERO_INT
  Byte_2 : Subsystem
  Byte_3 : Subsystem
  Byte_4 : Subsystem
  Byte_5 : Subsystem
  Byte_6 : Subsystem
  Byte_7 : Subsystem
  CAASSta : Subsystem
  CRC8_IfAction_Tx : Subsystem  AncestorBlock=FVT_lib/hal/CRC8_IfAction_Tx
      mask help: MeasumentTrigerEvent
      mask Display: fprintf('CRC8_IfAction');
  Constant : Constant  Value=KHAL_CAN6FD6APS3E2E_flg
  Constant1 : Constant  Value=0xE5
  Constant2 : Constant  Value=0x86
  Constant3 : Constant  Value=KHAL_CAN6FD6APS3E2E_flg
  Constant4 : Constant  Value=KHAL_CAN6FD6APS3E2E_flg
  Ground{,1..11} (12 alike) : Ground
  Mux2 : Mux  Inputs=15
  RollingCounter_IfAction : FVT_lib/hal/RollingCounter_IfAction
  RollingCounter_IfAction1 : FVT_lib/hal/RollingCounter_IfAction
  SPTGDet : Subsystem
  SPTGSta : Subsystem
  Terminator : Terminator
  bus_creator : BusCreator  Inputs=13  OutDataTypeStr=Bus: DT_CAN6_SG_FD6_APS3  NonVirtualBus=on
  bus_selector : BusSelector  OutputSignals=VOUTP_APSOpenPTG_flg
  bus_selector1 : BusSelector  OutputSignals=VOUTP_APSDecReqA_flg
  bus_selector10 : BusSelector  OutputSignals=VOUTP_APSStaSys_enum
  bus_selector11 : BusSelector  OutputSignals=VOUTP_SPTGDet_flg
  bus_selector2 : BusSelector  OutputSignals=VOUTP_APSReq_enum
  bus_selector3 : BusSelector  OutputSignals=VOUTP_APSDecReq_mps2
  bus_selector4 : BusSelector  OutputSignals=VOUTP_APSStaSys_enum
  bus_selector5 : BusSelector  OutputSignals=VOUTP_SPTGDet_flg
  bus_selector6 : BusSelector  OutputSignals=VOUTP_APSOpenPTG_flg
  bus_selector7 : BusSelector  OutputSignals=VOUTP_APSDecReq_mps2
  bus_selector8 : BusSelector  OutputSignals=VOUTP_APSDecReqA_flg
  bus_selector9 : BusSelector  OutputSignals=VOUTP_APSReq_enum
  FD6_APS3 : Outport
  wires:
  BSCP_outputs/1 -> [BSCP_outputs]
  BOUTP_outputs/1 -> [BOUTP_outputs]
  [CAN6_APS3_LifeCount] -> bus_creator/1  "CAN6_APS3_LifeCount"
  [CAN6_APS3_checksum] -> bus_creator/2  "CAN6_APS3_checksum"
  [CAN6_APSOpenPTG] -> bus_creator/3  "CAN6_APSOpenPTG"
  [CAN6_APS_Angle_Target] -> bus_creator/4  "CAN6_APS_Angle_Target"
  [CAN6_APS_DecReq] -> bus_creator/5  "CAN6_APS_DecReq"
  [CAN6_APS_DecReq_A] -> bus_creator/6  "CAN6_APS_DecReq_A"
  [CAN6_APS_Req] -> bus_creator/7  "CAN6_APS_Req"
  [CAN6_APS_Rq_EPS_Ctrl] -> bus_creator/8  "CAN6_APS_Rq_EPS_Ctrl"
  [CAN6_APS_Sta_System] -> bus_creator/9  "CAN6_APS_Sta_System"
  [CAN6_APS_V_Rq_EPS_Ctrl] -> bus_creator/10  "CAN6_APS_V_Rq_EPS_Ctrl"
  [CAN6_CAAS_Sta] -> bus_creator/11  "CAN6_CAAS_Sta"
  [CAN6_SPTGDet] -> bus_creator/12  "CAN6_SPTGDet"
  [CAN6_SPTG_Sta] -> bus_creator/13  "CAN6_SPTG_Sta"
  bus_creator/1 -> FD6_APS3/1
  APS3LifeCount/1(CAN6_APS3_LifeCount) -> [CAN6_APS3_LifeCount]
  APS3checksum/1(CAN6_APS3_checksum) -> [CAN6_APS3_checksum]
  APSOpenPTG/1(CAN6_APSOpenPTG) -> [CAN6_APSOpenPTG]
  APSAngleTarget/1(CAN6_APS_Angle_Target) -> [CAN6_APS_Angle_Target]
  APSDecReq/1(CAN6_APS_DecReq) -> [CAN6_APS_DecReq]
  APSDecReqA/1(CAN6_APS_DecReq_A) -> [CAN6_APS_DecReq_A]
  APSReq/1(CAN6_APS_Req) -> [CAN6_APS_Req]
  APSRqEPSCtrl/1(CAN6_APS_Rq_EPS_Ctrl) -> [CAN6_APS_Rq_EPS_Ctrl]
  APSStaSystem/1(CAN6_APS_Sta_System) -> [CAN6_APS_Sta_System]
  APSVRqEPSCtrl/1(CAN6_APS_V_Rq_EPS_Ctrl) -> [CAN6_APS_V_Rq_EPS_Ctrl]
  CAASSta/1(CAN6_CAAS_Sta) -> [CAN6_CAAS_Sta]
  SPTGDet/1(CAN6_SPTGDet) -> [CAN6_SPTGDet]
  SPTGSta/1(CAN6_SPTG_Sta) -> [CAN6_SPTG_Sta]
  Byte_0/1(Byte_0) -> Terminator/1
  Byte_1/1(Byte_1) -> [Byte_1]
  Byte_2/1(Byte_2) -> [Byte_2]
  Byte_3/1(Byte_3) -> [Byte_3]
  Byte_4/1(Byte_4) -> [Byte_4]
  Byte_5/1(Byte_5) -> [Byte_5]
  Byte_6/1(Byte_6) -> [Byte_6]
  Byte_7/1(Byte_7) -> [Byte_7]
  Byte_8/1 -> [Byte_8]
  Byte_9/1 -> [Byte_9]
  Byte_10/1 -> [Byte_10]
  Byte_11/1 -> [Byte_11]
  Byte_12/1 -> [Byte_12]
  Byte_13/1 -> [Byte_13]
  Byte_14/1 -> [Byte_14]
  Byte_15/1 -> [Byte_15]
  Mux2/1 -> CRC8_IfAction_Tx/4(RawData)
  Constant/1 -> CRC8_IfAction_Tx/1(CAN_E2E_flg)
  Constant1/1 -> CRC8_IfAction_Tx/2(DataID1)
  Constant2/1 -> CRC8_IfAction_Tx/3(DataID2)
  CRC8_IfAction_Tx/1(CRC8) -> [APS3_checksum]
  Ground/1 -> Byte_0/1(APS3_checksum)
  [Byte_1] -> Mux2/1
  RollingCounter_IfAction/1 -> Byte_1/1(APS3_LifeCount)
  Constant3/1 -> RollingCounter_IfAction/1
  [Byte_2] -> Mux2/2
  bus_selector/1 -> Byte_2/1(APSOpenPTG)  "<VOUTP_APSOpenPTG_flg>"
  [BOUTP_outputs] -> bus_selector/1
  bus_selector1/1 -> Byte_2/2(APS_DecReq_A)  "<VOUTP_APSDecReqA_flg>"
  [BOUTP_outputs] -> bus_selector1/1
  bus_selector2/1 -> Byte_2/3(APS_Req)  "<VOUTP_APSReq_enum>"
  [BOUTP_outputs] -> bus_selector2/1
  Ground1/1 -> Byte_2/4(CAAS_Sta)
  [Byte_3] -> Mux2/3
  bus_selector3/1 -> Byte_3/1(APS_DecReq)  "<VOUTP_APSDecReq_mps2>"
  [BOUTP_outputs] -> bus_selector3/1
  [Byte_4] -> Mux2/4
  Ground2/1 -> Byte_4/1(APS_Angle_Target)
  [Byte_5] -> Mux2/5
  Ground3/1 -> Byte_5/1(APS_Angle_Target)
  [Byte_6] -> Mux2/6
  bus_selector4/1 -> Byte_6/1(APS_Sta_System)  "<VOUTP_APSStaSys_enum>"
  [BOUTP_outputs] -> bus_selector4/1
  Ground4/1 -> Byte_6/2(APS_V_Rq_EPS_Ctrl)
  bus_selector5/1 -> Byte_6/3(SPTGDet)  "<VOUTP_SPTGDet_flg>"
  [BOUTP_outputs] -> bus_selector5/1
  Ground5/1 -> Byte_6/4(SPTG_Sta)
  [Byte_7] -> Mux2/7
  Ground6/1 -> Byte_7/1(APS_Rq_EPS_Ctrl)
  [Byte_8] -> Mux2/8
  [Byte_9] -> Mux2/9
  [Byte_10] -> Mux2/10
  [Byte_11] -> Mux2/11
  [Byte_12] -> Mux2/12
  [Byte_13] -> Mux2/13
  [Byte_14] -> Mux2/14
  [Byte_15] -> Mux2/15
  RollingCounter_IfAction1/1 -> APS3LifeCount/1(APS3LifeCount)
  Constant4/1 -> RollingCounter_IfAction1/1
  [APS3_checksum] -> APS3checksum/1(APS3checksum)
  bus_selector6/1 -> APSOpenPTG/1(APSOpenPTG)  "<VOUTP_APSOpenPTG_flg>"
  [BOUTP_outputs] -> bus_selector6/1
  Ground7/1 -> APSAngleTarget/1(APSAngleTarget)
  bus_selector7/1 -> APSDecReq/1(APSDecReq)  "<VOUTP_APSDecReq_mps2>"
  [BOUTP_outputs] -> bus_selector7/1
  bus_selector8/1 -> APSDecReqA/1(APSDecReqA)  "<VOUTP_APSDecReqA_flg>"
  [BOUTP_outputs] -> bus_selector8/1
  bus_selector9/1 -> APSReq/1(APSReq)  "<VOUTP_APSReq_enum>"
  [BOUTP_outputs] -> bus_selector9/1
  Ground8/1 -> APSRqEPSCtrl/1(APSRqEPSCtrl)
  bus_selector10/1 -> APSStaSystem/1(APSStaSystem)  "<VOUTP_APSStaSys_enum>"
  [BOUTP_outputs] -> bus_selector10/1
  Ground9/1 -> APSVRqEPSCtrl/1(APSVRqEPSCtrl)
  Ground10/1 -> CAASSta/1(CAASSta)
  bus_selector11/1 -> SPTGDet/1(SPTGDet)  "<VOUTP_SPTGDet_flg>"
  [BOUTP_outputs] -> bus_selector11/1
  Ground11/1 -> SPTGSta/1(SPTGSta)

== system halout/HAL_OUT/CAN6/FD6_APS3_Tx ==
  TxReq : Inport
  Chart : Stateflow chart  TreatAsAtomicUnit=on
  Constant : Constant  Value=C_TASK_5MS_S
  Constant3 : Constant  Value=CycleTime
  Data Type Conversion : DataTypeConversion  OutDataTypeStr=uint16
  Divide : Product  Inputs=*/
  Gain : Gain  Gain=0.001
  TxTrigger : Outport
  wires:
  Data Type Conversion/1 -> Chart/2(CycleCnt)
  Constant3/1 -> Gain/1
  Gain/1 -> Divide/1
  Chart/1(TxTrigger()) -> TxTrigger/1
  Divide/1 -> Data Type Conversion/1
  TxReq/1 -> Chart/1(TxReq)
  Constant/1 -> Divide/2
